simulink library "mqlib"  (R2024b)
settings: Solver=VariableStepAuto  StartTime=0.0  StopTime=10.0  RelTol=1e-3
undefined symbols (not defined in the file): DiscIntNeverNeededParam
settings Model: Creator=yangyu  LastModifiedBy=yangyu

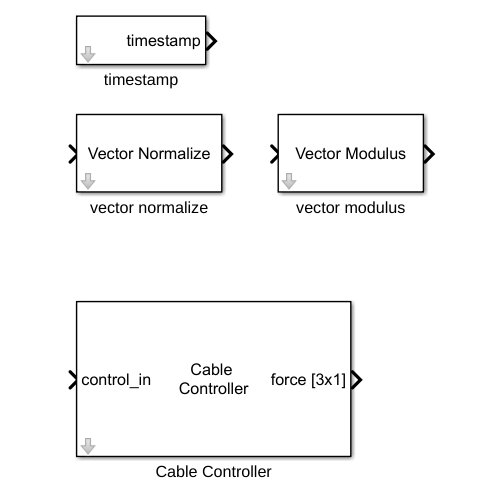
[thumbnail: Simulink's stored preview of the top-level diagram]
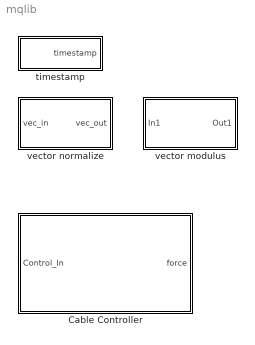
== system mqlib ==
  Cable Controller : Subsystem  mask{Kq=0, Kw=0, mi=0, li=0}
      mask DialogControl DescGroupVar Prompt: Cable Controller
      mask Display:
      | disp('Cable \nController');
      | 
      | port_label('input', 1, 'control_in');
      | port_label('output', 1, 'force [3x1]');
  timestamp : Subsystem
      mask DialogControl DescGroupVar Prompt: Timestamp
      mask DialogControl DescTextVar Prompt: Get the current system timestamp.
      mask Display: port_label('output', 1, 'timestamp');
  vector modulus : Subsystem
      mask Display: disp('Vector Modulus')
  vector normalize : Subsystem
      mask Display: disp('Vector Normalize');

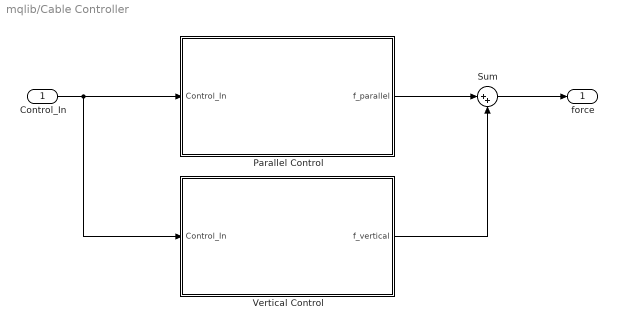
== system mqlib/Cable Controller ==
  Control_In : Inport  OutDataTypeStr=Bus: Control_In_Bus
  Parallel Control : Subsystem
  Sum : Sum  Inputs=|++
  Vertical Control : Subsystem
  force : Outport
  wires:
  Control_In/1 -> Vertical Control/1(Control_In), Parallel Control/1(Control_In)
  Vertical Control/1(f_vertical) -> Sum/2
  Parallel Control/1(f_parallel) -> Sum/1
  Sum/1 -> force/1

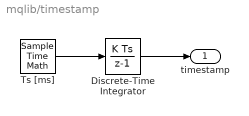
== system mqlib/timestamp ==
  Discrete-Time Integrator : DiscreteIntegrator  SampleTime=-1  OutDataTypeStr=Inherit: Inherit via back propagation  ICPrevOutput=DiscIntNeverNeededParam  ICPrevScaledInput=DiscIntNeverNeededParam
  Ts [ms] : SampleTimeMath  TsampMathOp=Ts Only  weightValue=1000  OutDataTypeStr=Inherit: Inherit via back propagation
  timestamp : Outport
  wires:
  Discrete-Time Integrator/1 -> timestamp/1
  Ts [ms]/1 -> Discrete-Time Integrator/1

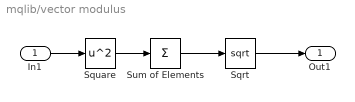
== system mqlib/vector modulus ==
  In1 : Inport
  Sqrt : Sqrt
  Square : Math  Operator=square
  Sum of Elements : Sum  Inputs=+
  Out1 : Outport
  wires:
  In1/1 -> Square/1
  Square/1 -> Sum of Elements/1
  Sum of Elements/1 -> Sqrt/1
  Sqrt/1 -> Out1/1

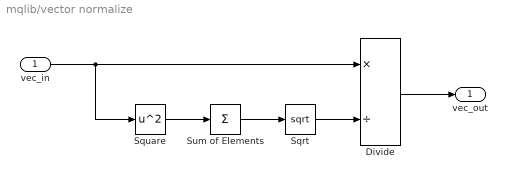
== system mqlib/vector normalize ==
  vec_in : Inport
  Divide : Product  Inputs=*/
  Sqrt : Sqrt
  Square : Math  Operator=square
  Sum of Elements : Sum  Inputs=+
  vec_out : Outport
  wires:
  Square/1 -> Sum of Elements/1
  Sum of Elements/1 -> Sqrt/1
  vec_in/1 -> Divide/1, Square/1
  Sqrt/1 -> Divide/2
  Divide/1 -> vec_out/1

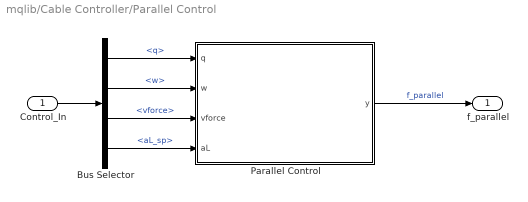
== system mqlib/Cable Controller/Parallel Control ==
  Control_In : Inport
  Bus Selector : BusSelector  OutputSignals=q,w,vforce,aL_sp
  Parallel Control : MATLAB Function  TreatAsAtomicUnit=on  mask{mi=mi, li=li}
  f_parallel : Outport
  wires:
  Bus Selector/4 -> Parallel Control/4(aL)  "<aL_sp>"
  Bus Selector/2 -> Parallel Control/2(w)  "<w>"
  Bus Selector/1 -> Parallel Control/1(q)  "<q>"
  Bus Selector/3 -> Parallel Control/3(vforce)  "<vforce>"
  Parallel Control/1(y) -> f_parallel/1  "f_parallel"
  Control_In/1 -> Bus Selector/1

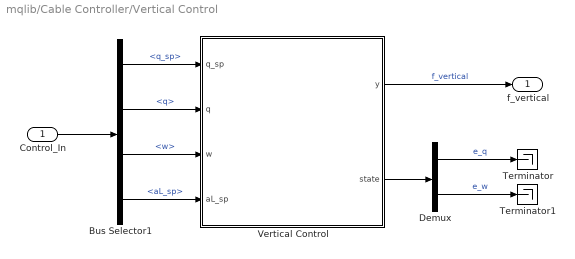
== system mqlib/Cable Controller/Vertical Control ==
  Control_In : Inport
  Bus Selector1 : BusSelector  OutputSignals=q_sp,q,w,aL_sp
  Demux : Demux  Outputs=2
  Terminator : Terminator
  Terminator1 : Terminator
  Vertical Control : MATLAB Function  TreatAsAtomicUnit=on  mask{mi=mi, li=li, Kq=Kq, Kw=Kw}
  f_vertical : Outport
  wires:
  Bus Selector1/1 -> Vertical Control/1(q_sp)  "<q_sp>"
  Bus Selector1/2 -> Vertical Control/2(q)  "<q>"
  Control_In/1 -> Bus Selector1/1
  Vertical Control/1(y) -> f_vertical/1  "f_vertical"
  Bus Selector1/3 -> Vertical Control/3(w)  "<w>"
  Bus Selector1/4 -> Vertical Control/4(aL_sp)  "<aL_sp>"
  Vertical Control/2(state) -> Demux/1
  Demux/1 -> Terminator/1  "e_q"
  Demux/2 -> Terminator1/1  "e_w"

== matlab function mqlib/Cable Controller/Parallel Control/Parallel Control ==
  data: q input; y output; w input; vforce input; aL input; mi parameter; li parameter
function y = fcn(q, w, vforce, aL, mi, li)

y = vforce * q + mi * li * (norm(w) ^ 2) * q + mi * q * q' * aL;

== matlab function mqlib/Cable Controller/Vertical Control/Vertical Control ==
  data: q_sp input; q input; w input; y output; aL_sp input; mi parameter; li parameter; Kq parameter; Kw parameter; state output
function [y, state] = fcn(q_sp, q, w, aL_sp, mi, li, Kq, Kw)
%% control law
Sqi = [0 -q(3) q(2); q(3) 0 -q(1); -q(2) q(1) 0];
e_q = cross(q_sp, q);
w_sp = -Kq * e_q;
e_w = w + Sqi * Sqi * w_sp;
y = mi * li * Sqi * (-Kw * e_w - Sqi * Sqi * w_sp) - mi * Sqi * Sqi * aL_sp;
%% record
state = [e_q; e_w] ;
